simulink model "IEEE14_case"  (R2024b)
settings: Solver=FixedStepAuto  StartTime=0  StopTime=2  FixedStep=1e-7  RelTol=1e-3
values from neighbouring files (symbols this model uses):
  GFL_15_Bva = 0.009    [IEEE14_parameters.m]
  GFL_15_C_bus_pu = 7.179419    [IEEE14_parameters.m]
  GFL_15_f0 = 60    [IEEE14_parameters.m]
  GFL_15_I_id = 691.26967    [IEEE14_parameters.m]
  GFL_15_I_iq = 691.26967    [IEEE14_parameters.m]
  GFL_15_I_od = 45.2207    [IEEE14_parameters.m]
  GFL_15_I_oq = 45.2207    [IEEE14_parameters.m]
  GFL_15_I_pll = 0.78    [IEEE14_parameters.m]
  GFL_15_Kdi = 0.09    [IEEE14_parameters.m]
  GFL_15_Kdo = 0.9    [IEEE14_parameters.m]
  GFL_15_Kqi = 0.09    [IEEE14_parameters.m]
  GFL_15_Kqo = 0.9    [IEEE14_parameters.m]
  GFL_15_Lg_pu = 0.631447    [IEEE14_parameters.m]
  GFL_15_mode = 1    [IEEE14_parameters.m]
  GFL_15_P_id = 3.7166    [IEEE14_parameters.m]
  GFL_15_P_iq = 3.7166    [IEEE14_parameters.m]
  GFL_15_P_od = 0.4798    [IEEE14_parameters.m]
  GFL_15_P_oq = 0.4798    [IEEE14_parameters.m]
  GFL_15_P_pll = 290.42    [IEEE14_parameters.m]
  GFL_15_Qe_ref = 0.2    [IEEE14_parameters.m]
  GFL_15_Rg_pu = 0.024016    [IEEE14_parameters.m]
  GFL_15_Sbase = 1.000000e+4    (= 10000)    [IEEE14_parameters.m]
  GFL_15_Tdi = 0.01    [IEEE14_parameters.m]
  GFL_15_Tdo = 0.2    [IEEE14_parameters.m]
  GFL_15_Tqi = 0.01    [IEEE14_parameters.m]
  GFL_15_Tqo = 0.2    [IEEE14_parameters.m]
  GFL_15_Vbase = 380    [IEEE14_parameters.m]
  GFL_15_Vdc_ref = 1.011475    [IEEE14_parameters.m]
  GFL_15_Vdcbase = 700    [IEEE14_parameters.m]
  GFL_15_vq_ref = 0    [IEEE14_parameters.m]
  GFL_16_Bva = 0.002    [IEEE14_parameters.m]
  GFL_16_C_bus_pu = 7.179419    [IEEE14_parameters.m]
  GFL_16_f0 = 60    [IEEE14_parameters.m]
  GFL_16_I_id = 691.26967    [IEEE14_parameters.m]
  GFL_16_I_iq = 691.26967    [IEEE14_parameters.m]
  GFL_16_I_od = 45.2207    [IEEE14_parameters.m]
  GFL_16_I_oq = 45.2207    [IEEE14_parameters.m]
  GFL_16_I_pll = 0.78    [IEEE14_parameters.m]
  GFL_16_Kdi = 0.05    [IEEE14_parameters.m]
  GFL_16_Kdo = 0.5    [IEEE14_parameters.m]
  GFL_16_Kqi = 0.05    [IEEE14_parameters.m]
  GFL_16_Kqo = 0.5    [IEEE14_parameters.m]
  GFL_16_Lg_pu = 0.631447    [IEEE14_parameters.m]
  GFL_16_mode = 1    [IEEE14_parameters.m]
  GFL_16_P_id = 3.7166    [IEEE14_parameters.m]
  GFL_16_P_iq = 3.7166    [IEEE14_parameters.m]
  GFL_16_P_od = 0.4798    [IEEE14_parameters.m]
  GFL_16_P_oq = 0.4798    [IEEE14_parameters.m]
  GFL_16_P_pll = 290.42    [IEEE14_parameters.m]
  GFL_16_Qe_ref = 0.2    [IEEE14_parameters.m]
  GFL_16_Rg_pu = 0.024016    [IEEE14_parameters.m]
  GFL_16_Sbase = 1.000000e+4    (= 10000)    [IEEE14_parameters.m]
  GFL_16_Tdi = 0.01    [IEEE14_parameters.m]
  GFL_16_Tdo = 0.2    [IEEE14_parameters.m]
  GFL_16_Tqi = 0.01    [IEEE14_parameters.m]
  GFL_16_Tqo = 0.2    [IEEE14_parameters.m]
  GFL_16_Vbase = 380    [IEEE14_parameters.m]
  GFL_16_Vdc_ref = 1.01144    [IEEE14_parameters.m]
  GFL_16_Vdcbase = 700    [IEEE14_parameters.m]
  GFL_16_vq_ref = 0    [IEEE14_parameters.m]
  GFL_17_Bva = 0.002    [IEEE14_parameters.m]
  GFL_17_C_bus_pu = 7.179419    [IEEE14_parameters.m]
  GFL_17_f0 = 60    [IEEE14_parameters.m]
  GFL_17_I_id = 691.26967    [IEEE14_parameters.m]
  GFL_17_I_iq = 691.26967    [IEEE14_parameters.m]
  GFL_17_I_od = 45.2207    [IEEE14_parameters.m]
  GFL_17_I_oq = 45.2207    [IEEE14_parameters.m]
  GFL_17_I_pll = 0.78    [IEEE14_parameters.m]
  GFL_17_Kdi = 0.05    [IEEE14_parameters.m]
  GFL_17_Kdo = 0.5    [IEEE14_parameters.m]
  GFL_17_Kqi = 0.05    [IEEE14_parameters.m]
  GFL_17_Kqo = 0.5    [IEEE14_parameters.m]
  GFL_17_Lg_pu = 0.631447    [IEEE14_parameters.m]
  GFL_17_mode = 1    [IEEE14_parameters.m]
  GFL_17_P_id = 3.7166    [IEEE14_parameters.m]
  GFL_17_P_iq = 3.7166    [IEEE14_parameters.m]
  GFL_17_P_od = 0.4798    [IEEE14_parameters.m]
  GFL_17_P_oq = 0.4798    [IEEE14_parameters.m]
  GFL_17_P_pll = 290.42    [IEEE14_parameters.m]
  GFL_17_Qe_ref = 0.2    [IEEE14_parameters.m]
  GFL_17_Rg_pu = 0.024016    [IEEE14_parameters.m]
  GFL_17_Sbase = 1.000000e+4    (= 10000)    [IEEE14_parameters.m]
  GFL_17_Tdi = 0.01    [IEEE14_parameters.m]
  GFL_17_Tdo = 0.2    [IEEE14_parameters.m]
  GFL_17_Tqi = 0.01    [IEEE14_parameters.m]
  GFL_17_Tqo = 0.2    [IEEE14_parameters.m]
  GFL_17_Vbase = 380    [IEEE14_parameters.m]
  GFL_17_Vdc_ref = 1.011632    [IEEE14_parameters.m]
  GFL_17_Vdcbase = 700    [IEEE14_parameters.m]
  GFL_17_vq_ref = 0    [IEEE14_parameters.m]
  GFL_18_Bva = 0.002    [IEEE14_parameters.m]
  GFL_18_C_bus_pu = 7.179419    [IEEE14_parameters.m]
  GFL_18_f0 = 60    [IEEE14_parameters.m]
  GFL_18_I_id = 691.26967    [IEEE14_parameters.m]
  GFL_18_I_iq = 691.26967    [IEEE14_parameters.m]
  GFL_18_I_od = 45.2207    [IEEE14_parameters.m]
  GFL_18_I_oq = 45.2207    [IEEE14_parameters.m]
  GFL_18_I_pll = 0.78    [IEEE14_parameters.m]
  GFL_18_Kdi = 0.05    [IEEE14_parameters.m]
  GFL_18_Kdo = 0.5    [IEEE14_parameters.m]
  GFL_18_Kqi = 0.05    [IEEE14_parameters.m]
  GFL_18_Kqo = 0.5    [IEEE14_parameters.m]
  GFL_18_Lg_pu = 0.631447    [IEEE14_parameters.m]
  GFL_18_mode = 1    [IEEE14_parameters.m]
  GFL_18_P_id = 3.7166    [IEEE14_parameters.m]
  GFL_18_P_iq = 3.7166    [IEEE14_parameters.m]
  GFL_18_P_od = 0.4798    [IEEE14_parameters.m]
  GFL_18_P_oq = 0.4798    [IEEE14_parameters.m]
  GFL_18_P_pll = 290.42    [IEEE14_parameters.m]
  GFL_18_Qe_ref = 0.2    [IEEE14_parameters.m]
  GFL_18_Rg_pu = 0.024016    [IEEE14_parameters.m]
  GFL_18_Sbase = 1.000000e+4    (= 10000)    [IEEE14_parameters.m]
  GFL_18_Tdi = 0.01    [IEEE14_parameters.m]
  GFL_18_Tdo = 0.2    [IEEE14_parameters.m]
  GFL_18_Tqi = 0.01    [IEEE14_parameters.m]
  GFL_18_Tqo = 0.2    [IEEE14_parameters.m]
  GFL_18_Vbase = 380    [IEEE14_parameters.m]
  GFL_18_Vdc_ref = 1.011572    [IEEE14_parameters.m]
  GFL_18_Vdcbase = 700    [IEEE14_parameters.m]
  GFL_18_vq_ref = 0    [IEEE14_parameters.m]
  ... (+180 more)
(part 1 of 25)
settings Model: SimulationMode=accelerator  Creator=Greg  LastModifiedBy=Greg
settings DataIOCC: ReturnWorkspaceOutputs=off

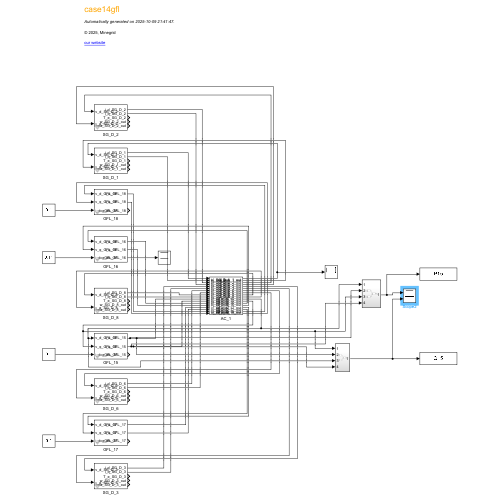
[thumbnail: Simulink's stored preview of the top-level diagram]
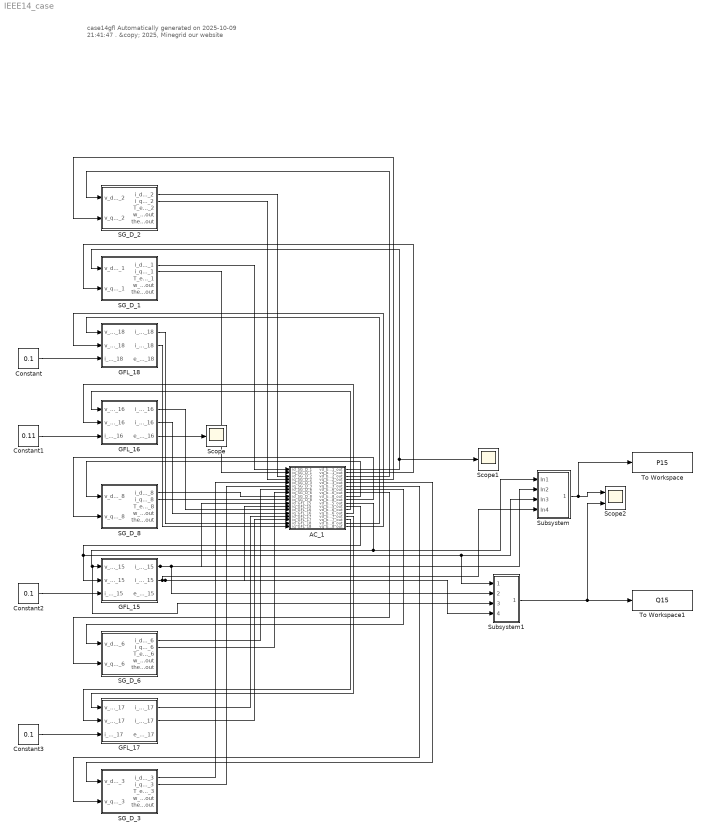
== system IEEE14_case ==
  note: case14gfl
      | Automatically generated on 2025-10-09 21:41:47 .
      | &copy; 2025, Minegrid
      | our website
  AC_1 : Subsystem  mask(AC_1){}
      mask help: Parameters Interface of AC_1
  Constant : Constant  Value=0.1
  Constant1 : Constant  Value=0.11
  Constant2 : Constant  Value=0.1
  Constant3 : Constant  Value=0.1
  GFL_15 : Subsystem  mask(GFL_15){Qe_ref=GFL_15_Qe_ref, Vdc_ref=GFL_15_Vdc_ref, mode=GFL_15_mode, C_bus_pu=GFL_15_C_bus_pu, Rg_pu=GFL_15_Rg_pu, Lg_pu=GFL_15_Lg_pu, P_od=GFL_15_P_od, I_od=GFL_15_I_od, P_oq=GFL_15_P_oq, I_oq=GFL_15_I_oq, P_id=GFL_15_P_id, I_id=GFL_15_I_id, P_iq=GFL_15_P_iq, I_iq=GFL_15_I_iq, P_pll=GFL_15_P_pll, I_pll=GFL_15_I_pll, f0=GFL_15_f0, Sbase=GFL_15_Sbase, Vbase=GFL_15_Vbase, Vdcbase=GFL_15_Vdcbase, vq_ref=GFL_15_vq_ref, Bva=GFL_15_Bva, Tdo=GFL_15_Tdo, Tdi=GFL_15_Tdi, Tqo=GFL_15_Tqo, Tqi=GFL_15_Tqi, Kdo=GFL_15_Kdo, Kdi=GFL_15_Kdi, Kqo=GFL_15_Kqo, Kqi=GFL_15_Kqi}
      mask help: Parameters Interface of GFL_15
  GFL_16 : Subsystem  mask(GFL_16){Qe_ref=GFL_16_Qe_ref, Vdc_ref=GFL_16_Vdc_ref, mode=GFL_16_mode, C_bus_pu=GFL_16_C_bus_pu, Rg_pu=GFL_16_Rg_pu, Lg_pu=GFL_16_Lg_pu, P_od=GFL_16_P_od, I_od=GFL_16_I_od, P_oq=GFL_16_P_oq, I_oq=GFL_16_I_oq, P_id=GFL_16_P_id, I_id=GFL_16_I_id, P_iq=GFL_16_P_iq, I_iq=GFL_16_I_iq, P_pll=GFL_16_P_pll, I_pll=GFL_16_I_pll, f0=GFL_16_f0, Sbase=GFL_16_Sbase, Vbase=GFL_16_Vbase, Vdcbase=GFL_16_Vdcbase, vq_ref=GFL_16_vq_ref, Bva=GFL_16_Bva, Tdo=GFL_16_Tdo, Tdi=GFL_16_Tdi, Tqo=GFL_16_Tqo, Tqi=GFL_16_Tqi, Kdo=GFL_16_Kdo, Kdi=GFL_16_Kdi, Kqo=GFL_16_Kqo, Kqi=GFL_16_Kqi}
      mask help: Parameters Interface of GFL_16
  GFL_17 : Subsystem  mask(GFL_17){Qe_ref=GFL_17_Qe_ref, Vdc_ref=GFL_17_Vdc_ref, mode=GFL_17_mode, C_bus_pu=GFL_17_C_bus_pu, Rg_pu=GFL_17_Rg_pu, Lg_pu=GFL_17_Lg_pu, P_od=GFL_17_P_od, I_od=GFL_17_I_od, P_oq=GFL_17_P_oq, I_oq=GFL_17_I_oq, P_id=GFL_17_P_id, I_id=GFL_17_I_id, P_iq=GFL_17_P_iq, I_iq=GFL_17_I_iq, P_pll=GFL_17_P_pll, I_pll=GFL_17_I_pll, f0=GFL_17_f0, Sbase=GFL_17_Sbase, Vbase=GFL_17_Vbase, Vdcbase=GFL_17_Vdcbase, vq_ref=GFL_17_vq_ref, Bva=GFL_17_Bva, Tdo=GFL_17_Tdo, Tdi=GFL_17_Tdi, Tqo=GFL_17_Tqo, Tqi=GFL_17_Tqi, Kdo=GFL_17_Kdo, Kdi=GFL_17_Kdi, Kqo=GFL_17_Kqo, Kqi=GFL_17_Kqi}
      mask help: Parameters Interface of GFL_17
  GFL_18 : Subsystem  mask(GFL_18){Qe_ref=GFL_18_Qe_ref, Vdc_ref=GFL_18_Vdc_ref, mode=GFL_18_mode, C_bus_pu=GFL_18_C_bus_pu, Rg_pu=GFL_18_Rg_pu, Lg_pu=GFL_18_Lg_pu, P_od=GFL_18_P_od, I_od=GFL_18_I_od, P_oq=GFL_18_P_oq, I_oq=GFL_18_I_oq, P_id=GFL_18_P_id, I_id=GFL_18_I_id, P_iq=GFL_18_P_iq, I_iq=GFL_18_I_iq, P_pll=GFL_18_P_pll, I_pll=GFL_18_I_pll, f0=GFL_18_f0, Sbase=GFL_18_Sbase, Vbase=GFL_18_Vbase, Vdcbase=GFL_18_Vdcbase, vq_ref=GFL_18_vq_ref, Bva=GFL_18_Bva, Tdo=GFL_18_Tdo, Tdi=GFL_18_Tdi, Tqo=GFL_18_Tqo, Tqi=GFL_18_Tqi, Kdo=GFL_18_Kdo, Kdi=GFL_18_Kdi, Kqo=GFL_18_Kqo, Kqi=GFL_18_Kqi}
      mask help: Parameters Interface of GFL_18
  SG_D_1 : Subsystem  mask(SG_D_1){T_0=SG_D_1_T_0, w_ref=SG_D_1_w_ref, V_ref=SG_D_1_V_ref, x_d=SG_D_1_x_d, x_dd=SG_D_1_x_dd, x_ddd=SG_D_1_x_ddd, x_q=SG_D_1_x_q, x_qd=SG_D_1_x_qd, x_qdd=SG_D_1_x_qdd, x_l=SG_D_1_x_l, R_a=SG_D_1_R_a, T_dd=SG_D_1_T_dd, T_ddd=SG_D_1_T_ddd, T_qd=SG_D_1_T_qd, T_qdd=SG_D_1_T_qdd, H=SG_D_1_H, D=SG_D_1_D, SpeedPara=SG_D_1_SpeedPara, K_A=SG_D_1_K_A, EnableSaturation=SG_D_1_EnableSaturation, f0=SG_D_1_f0, T_speed=SG_D_1_T_speed, T_E=SG_D_1_T_E, T_A=SG_D_1_T_A, T_F=SG_D_1_T_F, K_E=SG_D_1_K_E, K_F=SG_D_1_K_F, K_s=SG_D_1_K_s, T_1=SG_D_1_T_1, T_2=SG_D_1_T_2, T_3=SG_D_1_T_3, T_4=SG_D_1_T_4, T_w=SG_D_1_T_w, S_A=SG_D_1_S_A, S_B=SG_D_1_S_B, S_N=SG_D_1_S_N}
      mask help: Parameters Interface of SG_D_1
  SG_D_2 : Subsystem  mask(SG_D_2){T_0=SG_D_2_T_0, w_ref=SG_D_2_w_ref, V_ref=SG_D_2_V_ref, x_d=SG_D_2_x_d, x_dd=SG_D_2_x_dd, x_ddd=SG_D_2_x_ddd, x_q=SG_D_2_x_q, x_qd=SG_D_2_x_qd, x_qdd=SG_D_2_x_qdd, x_l=SG_D_2_x_l, R_a=SG_D_2_R_a, T_dd=SG_D_2_T_dd, T_ddd=SG_D_2_T_ddd, T_qd=SG_D_2_T_qd, T_qdd=SG_D_2_T_qdd, H=SG_D_2_H, D=SG_D_2_D, SpeedPara=SG_D_2_SpeedPara, K_A=SG_D_2_K_A, EnableSaturation=SG_D_2_EnableSaturation, f0=SG_D_2_f0, T_speed=SG_D_2_T_speed, T_E=SG_D_2_T_E, T_A=SG_D_2_T_A, T_F=SG_D_2_T_F, K_E=SG_D_2_K_E, K_F=SG_D_2_K_F, K_s=SG_D_2_K_s, T_1=SG_D_2_T_1, T_2=SG_D_2_T_2, T_3=SG_D_2_T_3, T_4=SG_D_2_T_4, T_w=SG_D_2_T_w, S_A=SG_D_2_S_A, S_B=SG_D_2_S_B, S_N=SG_D_2_S_N}
      mask help: Parameters Interface of SG_D_2
  SG_D_3 : Subsystem  mask(SG_D_3){T_0=SG_D_3_T_0, w_ref=SG_D_3_w_ref, V_ref=SG_D_3_V_ref, x_d=SG_D_3_x_d, x_dd=SG_D_3_x_dd, x_ddd=SG_D_3_x_ddd, x_q=SG_D_3_x_q, x_qd=SG_D_3_x_qd, x_qdd=SG_D_3_x_qdd, x_l=SG_D_3_x_l, R_a=SG_D_3_R_a, T_dd=SG_D_3_T_dd, T_ddd=SG_D_3_T_ddd, T_qd=SG_D_3_T_qd, T_qdd=SG_D_3_T_qdd, H=SG_D_3_H, D=SG_D_3_D, SpeedPara=SG_D_3_SpeedPara, K_A=SG_D_3_K_A, EnableSaturation=SG_D_3_EnableSaturation, f0=SG_D_3_f0, T_speed=SG_D_3_T_speed, T_E=SG_D_3_T_E, T_A=SG_D_3_T_A, T_F=SG_D_3_T_F, K_E=SG_D_3_K_E, K_F=SG_D_3_K_F, K_s=SG_D_3_K_s, T_1=SG_D_3_T_1, T_2=SG_D_3_T_2, T_3=SG_D_3_T_3, T_4=SG_D_3_T_4, T_w=SG_D_3_T_w, S_A=SG_D_3_S_A, S_B=SG_D_3_S_B, S_N=SG_D_3_S_N}
      mask help: Parameters Interface of SG_D_3
  SG_D_6 : Subsystem  mask(SG_D_6){T_0=SG_D_6_T_0, w_ref=SG_D_6_w_ref, V_ref=SG_D_6_V_ref, x_d=SG_D_6_x_d, x_dd=SG_D_6_x_dd, x_ddd=SG_D_6_x_ddd, x_q=SG_D_6_x_q, x_qd=SG_D_6_x_qd, x_qdd=SG_D_6_x_qdd, x_l=SG_D_6_x_l, R_a=SG_D_6_R_a, T_dd=SG_D_6_T_dd, T_ddd=SG_D_6_T_ddd, T_qd=SG_D_6_T_qd, T_qdd=SG_D_6_T_qdd, H=SG_D_6_H, D=SG_D_6_D, SpeedPara=SG_D_6_SpeedPara, K_A=SG_D_6_K_A, EnableSaturation=SG_D_6_EnableSaturation, f0=SG_D_6_f0, T_speed=SG_D_6_T_speed, T_E=SG_D_6_T_E, T_A=SG_D_6_T_A, T_F=SG_D_6_T_F, K_E=SG_D_6_K_E, K_F=SG_D_6_K_F, K_s=SG_D_6_K_s, T_1=SG_D_6_T_1, T_2=SG_D_6_T_2, T_3=SG_D_6_T_3, T_4=SG_D_6_T_4, T_w=SG_D_6_T_w, S_A=SG_D_6_S_A, S_B=SG_D_6_S_B, S_N=SG_D_6_S_N}
      mask help: Parameters Interface of SG_D_6
  SG_D_8 : Subsystem  mask(SG_D_8){T_0=SG_D_8_T_0, w_ref=SG_D_8_w_ref, V_ref=SG_D_8_V_ref, x_d=SG_D_8_x_d, x_dd=SG_D_8_x_dd, x_ddd=SG_D_8_x_ddd, x_q=SG_D_8_x_q, x_qd=SG_D_8_x_qd, x_qdd=SG_D_8_x_qdd, x_l=SG_D_8_x_l, R_a=SG_D_8_R_a, T_dd=SG_D_8_T_dd, T_ddd=SG_D_8_T_ddd, T_qd=SG_D_8_T_qd, T_qdd=SG_D_8_T_qdd, H=SG_D_8_H, D=SG_D_8_D, SpeedPara=SG_D_8_SpeedPara, K_A=SG_D_8_K_A, EnableSaturation=SG_D_8_EnableSaturation, f0=SG_D_8_f0, T_speed=SG_D_8_T_speed, T_E=SG_D_8_T_E, T_A=SG_D_8_T_A, T_F=SG_D_8_T_F, K_E=SG_D_8_K_E, K_F=SG_D_8_K_F, K_s=SG_D_8_K_s, T_1=SG_D_8_T_1, T_2=SG_D_8_T_2, T_3=SG_D_8_T_3, T_4=SG_D_8_T_4, T_w=SG_D_8_T_w, S_A=SG_D_8_S_A, S_B=SG_D_8_S_B, S_N=SG_D_8_S_N}
      mask help: Parameters Interface of SG_D_8
  Scope : Scope
  Scope1 : Scope
  Scope2 : Scope  NumInputPorts=2
  Subsystem : Subsystem
  Subsystem1 : Subsystem
  To Workspace : ToWorkspace  VariableName=P15  SampleTime=-1
  To Workspace1 : ToWorkspace  VariableName=Q15  SampleTime=-1
  wires:
  AC_1/5(vd_bus_3_out) -> SG_D_3/1(v_d_SG_D_3)
  AC_1/3(vd_bus_2_out) -> SG_D_2/1(v_d_SG_D_2)
  SG_D_2/1(i_d_SG_D_2) -> AC_1/3(id_SG_D_2)
  AC_1/2(vq_bus_1_out) -> SG_D_1/2(v_q_SG_D_1)
  SG_D_1/2(i_q_SG_D_1) -> AC_1/2(iq_SG_D_1)
  SG_D_1/1(i_d_SG_D_1) -> AC_1/1(id_SG_D_1)
  SG_D_2/2(i_q_SG_D_2) -> AC_1/4(iq_SG_D_2)
  GFL_15/2(i_q_GFL_15) -> Subsystem/4(In4), Subsystem1/4(In4), AC_1/12(iq_GFL_15)
  GFL_18/1(i_d_GFL_18) -> AC_1/17(id_GFL_18)
  GFL_18/2(i_q_GFL_18) -> AC_1/18(iq_GFL_18)
  SG_D_3/1(i_d_SG_D_3) -> AC_1/5(id_SG_D_3)
  GFL_16/1(i_d_GFL_16) -> AC_1/13(id_GFL_16)
  GFL_16/2(i_q_GFL_16) -> AC_1/14(iq_GFL_16)
  SG_D_8/1(i_d_SG_D_8) -> AC_1/9(id_SG_D_8)
  SG_D_8/2(i_q_SG_D_8) -> AC_1/10(iq_SG_D_8)
  GFL_15/1(i_d_GFL_15) -> Subsystem/2(In2), Subsystem1/2(In2), AC_1/11(id_GFL_15)
  AC_1/13(vd_bus_16_out) -> GFL_16/1(v_d_GFL_16)
  AC_1/11(vd_bus_15_out) -> Subsystem1/3(In3), GFL_15/1(v_d_GFL_15), Subsystem/1(In1)
  SG_D_6/1(i_d_SG_D_6) -> AC_1/7(id_SG_D_6)
  AC_1/9(vd_bus_8_out) -> SG_D_8/1(v_d_SG_D_8)
  SG_D_6/2(i_q_SG_D_6) -> AC_1/8(iq_SG_D_6)
  GFL_17/1(i_d_GFL_17) -> AC_1/15(id_GFL_17)
  GFL_17/2(i_q_GFL_17) -> AC_1/16(iq_GFL_17)
  SG_D_3/2(i_q_SG_D_3) -> AC_1/6(iq_SG_D_3)
  AC_1/1(vd_bus_1_out) -> Scope1/1, SG_D_1/1(v_d_SG_D_1)
  AC_1/4(vq_bus_2_out) -> SG_D_2/2(v_q_SG_D_2)
  AC_1/6(vq_bus_3_out) -> SG_D_3/2(v_q_SG_D_3)
  AC_1/7(vd_bus_6_out) -> SG_D_6/1(v_d_SG_D_6)
  AC_1/10(vq_bus_8_out) -> SG_D_8/2(v_q_SG_D_8)
  AC_1/8(vq_bus_6_out) -> SG_D_6/2(v_q_SG_D_6)
  AC_1/14(vq_bus_16_out) -> GFL_16/2(v_q_GFL_16)
  AC_1/15(vd_bus_17_out) -> GFL_17/1(v_d_GFL_17)
  AC_1/18(vq_bus_18_out) -> GFL_18/2(v_q_GFL_18)
  AC_1/16(vq_bus_17_out) -> GFL_17/2(v_q_GFL_17)
  AC_1/17(vd_bus_18_out) -> GFL_18/1(v_d_GFL_18)
  Constant/1 -> GFL_18/3(i_dc_GFL_18)
  Constant1/1 -> GFL_16/3(i_dc_GFL_16)
  Constant2/1 -> GFL_15/3(i_dc_GFL_15)
  Constant3/1 -> GFL_17/3(i_dc_GFL_17)
  GFL_16/3(e_dc_GFL_16) -> Scope/1
  AC_1/12(vq_bus_15_out) -> Subsystem/3(In3), Subsystem1/1(In1), GFL_15/2(v_q_GFL_15)
  Subsystem/1(Out1) -> To Workspace/1, Scope2/1
  Subsystem1/1(Out1) -> To Workspace1/1, Scope2/2
